simulink model "ABB_Samistar"  (R2020b)
settings: Solver=VariableStepAuto  StartTime=0.0  StopTime=50  RelTol=1e-3
model workspace (MAT data in the model file):
  KPS = Simulink.Parameter
  KPS.Value = 1
  KPS.DataType = 'auto'
  KPS.Dimensions = [1 1]
  KPU = Simulink.Parameter
  KPU.Value = 0.04
  KPU.DataType = 'auto'
  KPU.Dimensions = [1 1]
  P_dyn_ampl = Simulink.Parameter
  P_dyn_ampl.Value = 54
  P_dyn_ampl.DataType = 'auto'
  P_dyn_ampl.Dimensions = [1 1]
  P_dyn_slip = Simulink.Parameter
  P_dyn_slip.Value = 0.79333
  P_dyn_slip.DataType = 'auto'
  P_dyn_slip.Dimensions = [1 1]
  TIS = Simulink.Parameter
  TIS.Value = 1
  TIS.DataType = 'auto'
  TIS.Dimensions = [1 1]
  aantal_keer_freq_sinus = 30
  amplitude_sinus = 1
  freq_sinus = 50
  gewenste_ampitude_fasesp = 326
libraries: powerlib x12
settings Model: ParameterArgumentNames=KPU  OrderedModelArguments=off  Creator=Tijl J  LastModifiedBy=Tijl J
settings SolverCC: ZeroCrossAlgorithm=Adaptive  AlgebraicLoopSolver=LineSearch
settings DebuggingCC: IgnoredZcDiagnostic=none

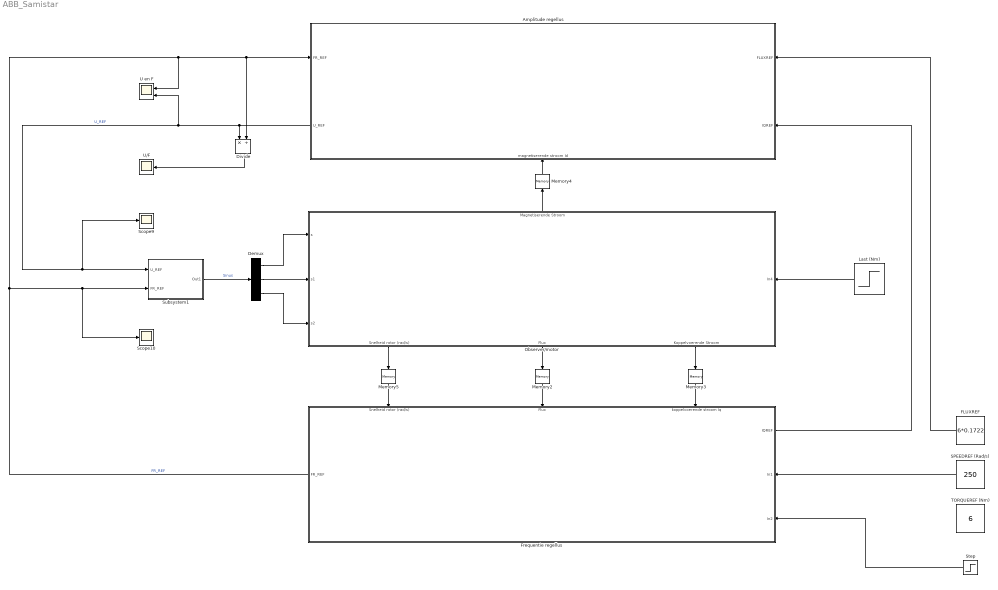
== system ABB_Samistar ==
  Amplitude regellus : Subsystem
      settings: PortSchema="{\"entries\":[{\"content\":{\"sides\":[{\"content\":{\"connectorIds\":[\"In1\",\"Out1\"]},\"type\":\"ConnectorPlacement.EquallySpacedRectSide\",\"uuid\":\"93bcf8db-9415-4baa-860c-11fdd531b56d\"},{\"content\":{\"connectorIds\":[\"In3\",\"In4\"],\"side\":\"RIGHT\"},\"type\":\"ConnectorPlacement.EquallySpacedRectSide\",\"uuid\":\"37029ce7-5e0f-4de3-a6e1-7a5c9d5a11f1\"},{\"content\":{\"connectorIds\":[],\"side\":\"TOP\"},\"type\":\"ConnectorPlacement.EquallySpacedRectSide\",\"uuid\":\"728afc0d-af0d-45f1-9722-28d57fd6c551\"},{\"content\":{\"connectorIds\":[\"In2\"],\"side\":\"BOTTOM\"},\"type\":\"ConnectorPlacement.EquallySpacedRectSide\",\"uuid\":\"07082ed3-f076-4bb5-ab11-0475c2dbd4ea\"}]},\"type\":\"ConnectorPlacement.EquallySpacedConnector\",\"uuid\":\"a9ce8458-6a15-4687-a7cd-fa30a873f563\"}],\"packageUris\":[\"http://schema.mathworks.com/mf0/Connector/19700101\"],\"version\":\"1.0\"}"
  Demux : Demux  Outputs=3
      settings: DisplayOption=none
  Divide : Product  Inputs=*/  RndMeth=Zero  SaturateOnIntegerOverflow=on
  FLUXREF : Constant  Value=6*0.1722
  Frequentie regellus : Subsystem
      settings: PortSchema="{\"entries\":[{\"content\":{\"sides\":[{\"content\":{\"connectorIds\":[\"Out2\"]},\"type\":\"ConnectorPlacement.EquallySpacedRectSide\",\"uuid\":\"9e8918ce-6ab1-4350-a27c-6c0740db8e36\"},{\"content\":{\"connectorIds\":[\"Out1\",\"In4\",\"In5\"],\"side\":\"RIGHT\"},\"type\":\"ConnectorPlacement.EquallySpacedRectSide\",\"uuid\":\"b7677f78-c4ce-4f8c-bcaa-757820ca5b4a\"},{\"content\":{\"connectorIds\":[\"In1\",\"In2\",\"In3\"],\"side\":\"TOP\"},\"type\":\"ConnectorPlacement.EquallySpacedRectSide\",\"uuid\":\"ce215d33-9ba4-4a26-b731-73f2d57ad5bf\"},{\"content\":{\"connectorIds\":[],\"side\":\"BOTTOM\"},\"type\":\"ConnectorPlacement.EquallySpacedRectSide\",\"uuid\":\"afaf8d9d-7f5b-47e6-9504-851e9c020fbe\"}]},\"type\":\"ConnectorPlacement.EquallySpacedConnector\",\"uuid\":\"a6238931-2ac8-4383-9bdd-f69522e27e3a\"}],\"packageUris\":[\"http://schema.mathworks.com/mf0/Connector/19700101\"],\"version\":\"1.0\"}"
  Last (Nm) : Step  Time=7  After=6  SampleTime=0
  Memory{2..5} (4 alike) : Memory
  Observer/motor : Subsystem
      settings: PortSchema="{\"entries\":[{\"content\":{\"sides\":[{\"content\":{\"connectorIds\":[\"In1\",\"In2\",\"In3\"]},\"type\":\"ConnectorPlacement.EquallySpacedRectSide\",\"uuid\":\"e974f17d-3e24-4aa3-9f71-ee26b6420732\"},{\"content\":{\"connectorIds\":[\"In4\"],\"side\":\"RIGHT\"},\"type\":\"ConnectorPlacement.EquallySpacedRectSide\",\"uuid\":\"7b407c95-e93c-432b-9353-b22fb20e7cb2\"},{\"content\":{\"connectorIds\":[\"Out4\"],\"side\":\"TOP\"},\"type\":\"ConnectorPlacement.EquallySpacedRectSide\",\"uuid\":\"82039074-d665-492a-9fb7-dc8321ceba23\"},{\"content\":{\"connectorIds\":[\"Out1\",\"Out2\",\"Out3\"],\"side\":\"BOTTOM\"},\"type\":\"ConnectorPlacement.EquallySpacedRectSide\",\"uuid\":\"28c56ceb-9a43-45d0-8e14-1b89590953e6\"}]},\"type\":\"ConnectorPlacement.EquallySpacedConnector\",\"uuid\":\"259d5e5a-eb05-4963-bbb5-562b18f45dd1\"}],\"packageUris\":[\"http://schema.mathworks.com/mf0/Connector/19700101\"],\"version\":\"1.0\"}"
  SPEEDREF (Rad/s) : Constant  Value=250
  Scope10 : Scope
  Scope9 : Scope
  Step : Step  Time=6  After=8  SampleTime=0
  Subsystem1 : Subsystem
  TORQUEREF (Nm) : Constant  Value=6
  U en F : Scope  NumInputPorts=2
  U/F : Scope
  wires:
  SPEEDREF (Rad/s)/1 -> Frequentie regellus/4(In1)
  FLUXREF/1 -> Amplitude regellus/3(FLUXREF)
  Frequentie regellus/1(IQREF) -> Amplitude regellus/4(IQREF)
  Amplitude regellus/1(U_REF) -> Scope9/1, Subsystem1/1(U_REF), U en F/2, Divide/1  "U_REF"
  Frequentie regellus/2(FR_REF) -> U en F/1, Amplitude regellus/1(FR_REF), Divide/2, Scope10/1, Subsystem1/2(FR_REF)  "FR_REF"
  Memory2/1 -> Frequentie regellus/2(Flux)
  Memory3/1 -> Frequentie regellus/3(koppelvoerende stroom Iq)
  Memory4/1 -> Amplitude regellus/2(magnetiserende stroom Id)
  Memory5/1 -> Frequentie regellus/1(Snelheid rotor (rad/s))
  Demux/1 -> Observer/motor/1(s)
  Demux/2 -> Observer/motor/2(s1)
  Demux/3 -> Observer/motor/3(s2)
  Observer/motor/4(Magnetiserende Stroom) -> Memory4/1
  Observer/motor/2(Flux) -> Memory2/1
  Observer/motor/1(Snelheid rotor (rad/s)) -> Memory5/1
  Observer/motor/3(Koppelvoerende Stroom) -> Memory3/1
  Subsystem1/1(Out1) -> Demux/1  "Sinus"
  Divide/1 -> U/F/1
  Last (Nm)/1 -> Observer/motor/4(In4)
  Step/1 -> Frequentie regellus/5(In2)

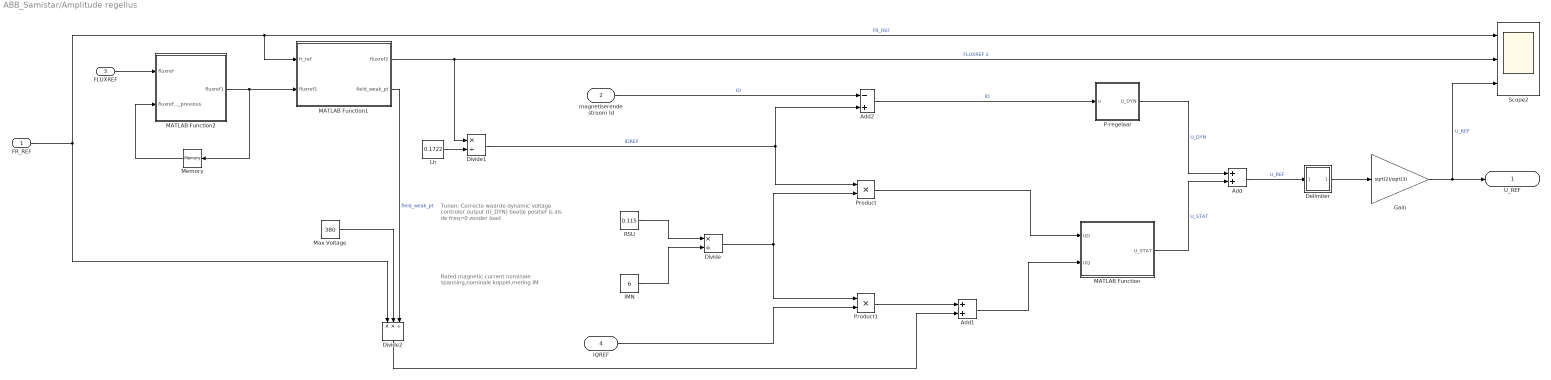
== system ABB_Samistar/Amplitude regellus ==
  note: Tunen:
      | Correcte waarde dynamic
      | voltage controler output (U_DYN)
      | beetje positief is als de freq=0 zonder load
  note: Rated magnetic current
      |
      | nominale spanning,nominale koppel,meting IM
  FR_REF : Inport
  magnetiserende stroom Id : Inport  Port=2
  FLUXREF : Inport  Port=3
  IQREF : Inport  Port=4
  Add : Sum
  Add1 : Sum
  Add2 : Sum  Inputs=-+
  Delimiter : MATLAB Function  TreatAsAtomicUnit=on
  Divide : Product  Inputs=*/
  Divide1 : Product  Inputs=*/
  Divide2 : Product  Inputs=**/
  Gain : Gain  Gain=sqrt(2)/sqrt(3)
  IMN : Constant  Value=6
  Lh : Constant  Value=0.1722
  MATLAB Function : MATLAB Function  TreatAsAtomicUnit=on
  MATLAB Function1 : MATLAB Function  TreatAsAtomicUnit=on  SystemSampleTime=0.001
  MATLAB Function2 : MATLAB Function  TreatAsAtomicUnit=on  SystemSampleTime=0.0001
  Max Voltage : Constant  Value=380
  Memory : Memory
  P-regelaar : Subsystem
  Product : Product
  Product1 : Product
  RSU : Constant  Value=0.115
  Scope2 : Scope  NumInputPorts=3
  U_REF : Outport
  wires:
  Add/1 -> Delimiter/1(U_REF_calculated)  "U_REF"
  MATLAB Function/1(U_STAT) -> Add/2  "U_STAT"
  Product/1 -> MATLAB Function/1(UD)
  Product1/1 -> Add1/1
  IQREF/1 -> Product1/2
  RSU/1 -> Divide/1
  IMN/1 -> Divide/2
  Divide/1 -> Product1/1, Product/2
  Add1/1 -> MATLAB Function/2(UQ)
  Divide2/1 -> Add1/2
  magnetiserende stroom Id/1 -> Add2/1  "ID"
  Divide1/1 -> Add2/2, Product/1  "IDREF"
  Add2/1 -> P-regelaar/1(u)  "ID"
  P-regelaar/1(U_DYN) -> Add/1  "U_DYN"
  MATLAB Function1/1(fluxref2) -> Divide1/1, Scope2/2  "FLUXREF 2"
  MATLAB Function2/1(fluxref1) -> Memory/1, MATLAB Function1/2(fluxref1)
  Memory/1 -> MATLAB Function2/2(fluxref1_previous)
  FR_REF/1 -> MATLAB Function1/1(fr_ref), Scope2/1, Divide2/1  "FR_REF"
  FLUXREF/1 -> MATLAB Function2/1(fluxref)
  MATLAB Function1/2(field_weak_pt) -> Divide2/3  "field_weak_pt"
  Max Voltage/1 -> Divide2/2
  Lh/1 -> Divide1/2
  Delimiter/1(U_REF) -> Gain/1
  Gain/1 -> U_REF/1, Scope2/3  "U_REF"

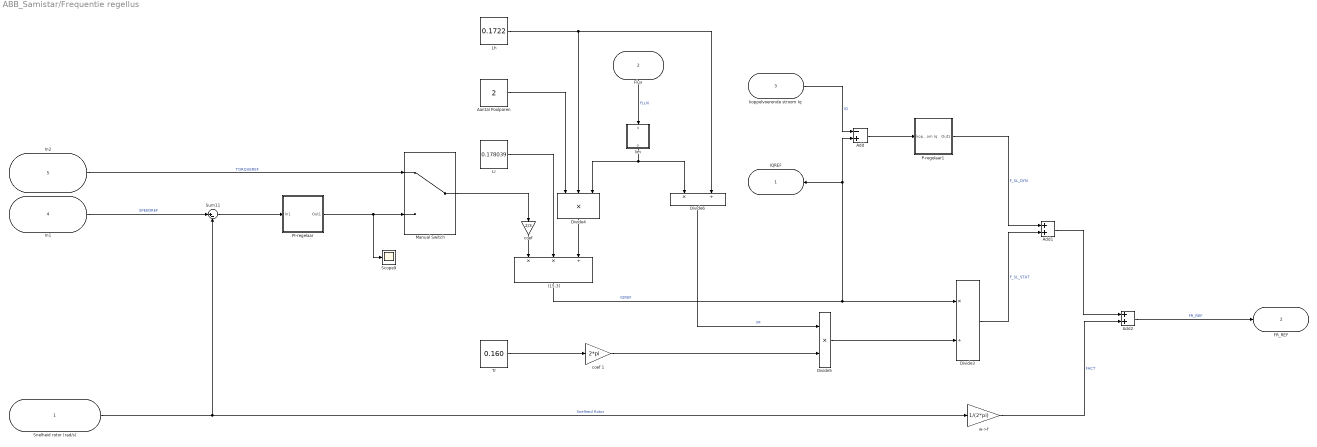
== system ABB_Samistar/Frequentie regellus ==
  Snelheid rotor (rad/s) : Inport
  Flux : Inport  Port=2
  koppelvoerende stroom Iq : Inport  Port=3
  In1 : Inport  Port=4
  In2 : Inport  Port=5
  (15.3) : Product  Inputs=**/
  Aantal Poolparen : Constant  Value=2
  Add : Sum  Inputs=-+
  Add1 : Sum
  Add2 : Sum
  Divide3 : Product  Inputs=*/
  Divide4 : Product  Inputs=***
  Divide5 : Product  Inputs=**
  Divide6 : Product  Inputs=*/
  Lh : Constant  Value=0.1722
  Lr : Constant  Value=0.178039
  Manual Switch : ManualSwitch
  P-regelaar1 : Subsystem
  PI-regelaar : Subsystem
  Scope9 : Scope
  Sum11 : Sum  Inputs=|+-
  Tr : Constant  Value=0.160
  "coef " : Gain  Gain=2/3
  coef 1 : Gain  Gain=2*pi
  lim : MATLAB Function  TreatAsAtomicUnit=on
  w->f : Gain  Gain=1/(2*pi)
  IQREF : Outport
  FR_REF : Outport  Port=2
  wires:
  Lh/1 -> Divide4/2, Divide6/2
  Divide4/1 -> (15.3)/3
  Aantal Poolparen/1 -> Divide4/1
  In2/1 -> Manual Switch/1  "TORQUEREF"
  Snelheid rotor (rad/s)/1 -> Sum11/2, w->f/1  "Snelheid Rotor"
  coef 1/1 -> Divide5/2
  Divide3/1 -> Add1/2  "F_SL_STAT"
  Sum11/1 -> PI-regelaar/1(In1)
  (15.3)/1 -> Add/2, IQREF/1, Divide3/1  "IQREF"
  PI-regelaar/1(Out1) -> Scope9/1, Manual Switch/2
  Flux/1 -> lim/1(u)  "FLUX"
  "coef "/1 -> (15.3)/1
  Add2/1 -> FR_REF/1  "FR_REF"
  Divide6/1 -> Divide5/1  "IM"
  Manual Switch/1 -> "coef "/1
  Tr/1 -> coef 1/1
  w->f/1 -> Add2/2  "FACT"
  P-regelaar1/1(Out1) -> Add1/1  "F_SL_DYN"
  Divide5/1 -> Divide3/2
  koppelvoerende stroom Iq/1 -> Add/1  "IQ"
  In1/1 -> Sum11/1  "SPEEDREF"
  Add/1 -> P-regelaar1/1(koppelvoerende stroom Iq)
  Lr/1 -> (15.3)/2
  lim/1(y) -> Divide6/1, Divide4/3
  Add1/1 -> Add2/1

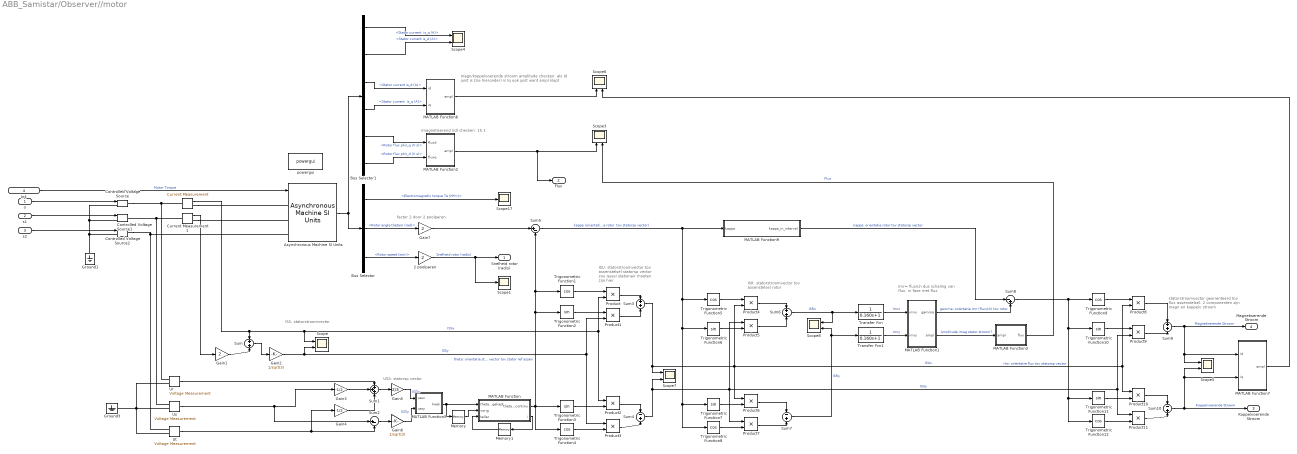
== system ABB_Samistar/Observer//motor ==
  note: Imagnetiserend (id) checken: 15.1
  note: magn/koppelvoerende stroom amplitude checken:
      | als Id juist is (zie hieronder) is Iq ook juist want ampl
      | klopt
  note: ISS: statorstroomvector
  note: USS: statorsp vector
  note: statorstroomvector georienteerd
      | tov flux assenstelsel: 2 componenten
      | zijn magn en koppelv stroom
  note: Imr= flux/Lh dus schaling
      | van flux, in fase met flux
  note: ISU: statorstroomvector tov
      | assenstelsel statorsp vector
      | zou quasi stationair moeten
      | zijn hier
  note: ISR: statorstroomvector tov
      | assenstelsel rotor
  note: factor 2 door 2 poolparen
  s : Inport
  s1 : Inport  Port=2
  s2 : Inport  Port=3
  In4 : Inport  Port=4
  " " : powerlib/Measurements/Current Measurement  PhasorSimulation=off  OutputType=Complex  PSBequivalent=0
  2 poolparen : Gain  Gain=2
  Asynchronous Machine SI Units : powerlib/Machines/Asynchronous Machine SI Units  RotorType=Squirrel-cage  PresetModel="15:  5.4 HP (4KW)   400 V  50Hz 1430 RPM"  MechanicalLoad=Torque Tm  ShowDetailedParameters=on  ReferenceFrame=Synchronous  Units=SI  MeasurementBus=off  NominalParameters=[4000 400 50]  Stator=[1.405 0.005839]  Rotor=[1.395 0.005839]  Cage1=[0.4155 0.002066]  Cage2=[0.4168 0.0003495]  Lm=0.1722  Mechanical=[0.0131 0.002985 2]  PolePairs=2  InitialConditions=[0 0 0 0 0 0 0 0]  SimulateSaturation=off  Saturation=[14.03593122, 27.81365428, 53.79336849, 68, 82, 96, 110,124, 130 ; 230, 322, 414, 460, 506, 552, 598, 644, 690]  LoadFlowParameters=1492000  TsPowergui=0  TsBlock=-1  IterativeModel=Trapezoidal non iterative  IterativeDiscreteModel=Trapezoidal non iterative  Pmec=1.492e+006
  Bus Selector : BusSelector  OutputSignals=Mechanical.Electromagnetic torque Te (N*m),Mechanical.Rotor angle thetam (rad),Mechanical.Rotor speed (wm)
  Bus Selector1 : BusSelector  OutputSignals="Stator measurements.Stator current  is_q (A),Stator measurements.Stator current is_d (A),Stator measurements.Stator current is_d (A),Stator measurements.Stator current  is_q (A),Rotor measurements.Rotor flux phir_q (V s),Rotor measurements.Rotor flux phir_d (V s)"
  Controlled Voltage Source : powerlib/Electrical Sources/Controlled Voltage Source  Initialize=on  Source_Type=AC  Amplitude=0  Phase=0  Frequency=0  Measurements=None
  Controlled Voltage Source1 : powerlib/Electrical Sources/Controlled Voltage Source  Initialize=on  Source_Type=AC  Amplitude=0  Phase=0  Frequency=0  Measurements=None
  Controlled Voltage Source2 : powerlib/Electrical Sources/Controlled Voltage Source  Initialize=on  Source_Type=AC  Amplitude=0  Phase=0  Frequency=0  Measurements=None
  Current Measurement1 : powerlib/Measurements/Current Measurement  PhasorSimulation=off  OutputType=Complex  PSBequivalent=0
  Gain1 : Gain  Gain=2
  Gain2 : Gain  Gain=1/sqrt(3)
  Gain3 : Gain  Gain=-1/2
  Gain4 : Gain  Gain=-1/2
  Gain5 : Gain  Gain=2/3
  Gain6 : Gain  Gain=1/sqrt(3)
  Gain7 : Gain  Gain=2
  Ground1 : powerlib/Elements/Ground  LConnTagsString=a
  Ground3 : powerlib/Elements/Ground  LConnTagsString=a
  MATLAB Function : MATLAB Function  TreatAsAtomicUnit=on
  MATLAB Function1 : MATLAB Function  TreatAsAtomicUnit=on
  MATLAB Function2 : MATLAB Function  TreatAsAtomicUnit=on
  MATLAB Function3 : MATLAB Function  TreatAsAtomicUnit=on
  MATLAB Function5 : MATLAB Function  TreatAsAtomicUnit=on
  MATLAB Function6 : MATLAB Function  TreatAsAtomicUnit=on
  MATLAB Function7 : MATLAB Function  TreatAsAtomicUnit=on
  MATLAB Function9 : MATLAB Function  TreatAsAtomicUnit=on
  Memory : Memory
  Memory1 : Memory
  Product{,1..11} (12 alike) : Product
  Scope{,3..8} (7 alike) : Scope  NumInputPorts=2
  Scope1 : Scope
  Scope17 : Scope
  Sum : Sum
  Sum1 : Sum  Inputs=3
  Sum10 : Sum  Inputs=-+
  Sum2 : Sum  Inputs=|+-
  Sum3 : Sum  Inputs=2
  Sum4 : Sum  Inputs=-+
  Sum5 : Sum  Inputs=|+-
  Sum6 : Sum
  Sum7 : Sum  Inputs=-+
  Sum8 : Sum  Inputs=|-+
  Sum9 : Sum
  Transfer Fcn : TransferFcn  Denominator=[0.160 1]
  Transfer Fcn1 : TransferFcn  Denominator=[0.160 1]
  Trigonometric Function{1,4..5,8..9,12} (6 alike) : Trigonometry  Operator=cos
  Trigonometric Function{2..3,6..7,10..11} (6 alike) : Trigonometry
  Ur : powerlib/Measurements/Voltage Measurement  PhasorSimulation=off  OutputType=Complex  PSBequivalent=0
  Us : powerlib/Measurements/Voltage Measurement  PhasorSimulation=off  OutputType=Complex  PSBequivalent=0
  Ut : powerlib/Measurements/Voltage Measurement  PhasorSimulation=off  OutputType=Complex  PSBequivalent=0
  powergui : powerlib/powergui  Priority=1  SimulationMode=Continuous  SampleTime=50e-6  frequency=60  Iterations=50  frequencyindice=50  Pbase=100e6  ErrMax=1e-4  UnitsV=kV  UnitsW=MW  buscounter=0  FunctionMessages=off  echomessages=off  EnableUseOfTLC=off  CurrentSourceSwitches=off  DisableSnubberDevices=off  DisableRonSwitches=off  DisableVfSwitches=off  DisplayEquations=off  AutomaticDiscreteSolvers=off  SolverType=Tustin/Backward Euler (TBE)  Interpol=off  ExternalGateDelay=off  methode=off  Ts=100  x0status=blocks  SPID=on  SwTol=0  HookPort=off  NonlinearTolerance=1e-4  nMaxIteration=100  ContinueOnMaxIteration=off  RestoreLinks=warning  ResistiveCurrentMeasurement=off  Frange=[0:2:500]  Ylog=off  Xlog=on  ShowGrid=off  save=off  variable=ZData  structure=0  ZoomFFT=off  StartTime=0.0  cycles=1  DisplayStyle=1  fundamental=60  FreqAxis=off  MaxFrequency=1000  frequencyindicesteady=1  RmsSteady=1  display=off
  Snelheid rotor (rad/s) : Outport
  Flux : Outport  Port=2
  Koppelvoerende Stroom : Outport  Port=3
  Magnetiserende Stroom : Outport  Port=4
  wires:
  Gain1/1 -> Sum/2
  Trigonometric Function8/1 -> Product7/2
  Ur/1 -> Sum1/1
  Product3/1 -> Sum4/2
  Bus Selector1/2 -> Scope4/2  "<Stator current is_d (A)>"
  Bus Selector/2 -> Gain7/1  "<Rotor angle thetam (rad)>"
  Asynchronous Machine SI Units/1 -> Bus Selector1/1, Bus Selector/1
  Bus Selector1/1 -> Scope4/1  "<Stator current  is_q (A)>"
  Us/1 -> Gain3/1, Sum2/1
  Sum8/1 -> Trigonometric Function12/1, Trigonometric Function11/1, Trigonometric Function10/1, Trigonometric Function9/1  "rho: oriëntatie flux tov statorsp vector"
  MATLAB Function/1(theta_continu) -> Trigonometric Function4/1, Trigonometric Function1/1, Sum5/2, Trigonometric Function2/1, Trigonometric Function3/1  "theta: orientatie stator sp vector tov stator ref assen"
  Product5/1 -> Sum6/2
  Trigonometric Function7/1 -> Product6/2
  s/1 -> Controlled Voltage Source/1
  Sum10/1 -> Scope5/2, MATLAB Function7/2(iq), Koppelvoerende Stroom/1  "Koppelvoerende Stroom"
  Sum4/1 -> Product11/1, Product9/2, Product5/1, Product7/1, Scope7/2  "ISUy"
  Trigonometric Function4/1 -> Product3/2
  Ut/1 -> Gain4/1, Sum2/2
  MATLAB Function2/1(ampl) -> Flux/1, Scope3/1
  Sum3/1 -> Product8/2, Product10/1, Product4/2, Product6/1, Scope7/1  "ISUx"
  Sum/1 -> Gain2/1
  Current Measurement1/1 -> Gain1/1
  Sum5/1 -> MATLAB Function9/1(kappa), Trigonometric Function8/1, Trigonometric Function7/1, Trigonometric Function6/1, Trigonometric Function5/1  "kappa (orientatie rotor  tov statorsp vector)"
  Trigonometric Function9/1 -> Product8/1
  MATLAB Function5/1(hoek) -> Memory/1, MATLAB Function/1(theta_gekapt)
  Sum1/1 -> Gain5/1
  Gain4/1 -> Sum1/3
  Gain7/1 -> Sum5/1
  Trigonometric Function2/1 -> Product1/1
  Product4/1 -> Sum6/1
  Gain5/1 -> MATLAB Function5/1(ussx)  "USSx"
  Product7/1 -> Sum7/2
  s2/1 -> Controlled Voltage Source2/1
  Sum2/1 -> Gain6/1
  Sum9/1 -> Scope5/1, MATLAB Function7/1(id), Magnetiserende Stroom/1  "Magnetiserende Stroom"
  MATLAB Function7/1(ampl) -> Scope6/2
  Sum6/1 -> Scope8/1, Transfer Fcn/1  "ISRx"
  MATLAB Function9/1(kappa_in_interval) -> Sum8/1  "kappa: orientatie rotor tov statorsp vector"
  Product/1 -> Sum3/1
  s1/1 -> Controlled Voltage Source1/1
  Trigonometric Function3/1 -> Product2/2
  Product1/1 -> Sum3/2
  2 poolparen/1 -> Scope1/1, Snelheid rotor (rad/s)/1  "Snelheid rotor (rad/s)"
  " "/1 -> Sum/1, Scope/1, Product/2, Product2/1  "ISSx"
  Gain2/1 -> Scope/2, Product1/2, Product3/1  "ISSy"
  MATLAB Function1/2(ampl) -> MATLAB Function3/1(ampl)  "Amplitude imag stator stroom?"
  Trigonometric Function6/1 -> Product5/2
  Product6/1 -> Sum7/1
  Gain6/1 -> MATLAB Function5/2(ussy)  "USSy"
  Trigonometric Function5/1 -> Product4/1
  Bus Selector/1 -> Scope17/1  "<Electromagnetic torque Te (N*m)>"
  Product2/1 -> Sum4/1
  Memory/1 -> MATLAB Function/2(vorig)
  Memory1/1 -> MATLAB Function/3(teller)
  MATLAB Function/2(i) -> Memory1/1
  Trigonometric Function10/1 -> Product9/1
  Sum7/1 -> Scope8/2, Transfer Fcn1/1  "ISRy"
  Product10/1 -> Sum10/1
  Product9/1 -> Sum9/2
  Trigonometric Function12/1 -> Product11/2
  Gain3/1 -> Sum1/2
  Trigonometric Function11/1 -> Product10/2
  Transfer Fcn/1 -> MATLAB Function1/1(imrx)  "Imrx"
  MATLAB Function1/1(gamma) -> Sum8/2  "gamma: oriëntatie Imr (flux/Lh) tov rotor"
  Bus Selector1/5 -> MATLAB Function2/1(fluxd)  "<Rotor flux phir_q (V s)>"
  Bus Selector1/3 -> MATLAB Function6/1(id)  "<Stator current is_d (A)>"
  Product8/1 -> Sum9/1
  MATLAB Function6/1(ampl) -> Scope6/1
  MATLAB Function3/1(flux) -> Scope3/2  "Flux"
  Trigonometric Function1/1 -> Product/1
  Bus Selector/3 -> 2 poolparen/1  "<Rotor speed (wm)>"
  Bus Selector1/4 -> MATLAB Function6/2(iq)  "<Stator current  is_q (A)>"
  Transfer Fcn1/1 -> MATLAB Function1/2(imry)  "Imry"
  Product11/1 -> Sum10/2
  Bus Selector1/6 -> MATLAB Function2/2(fluxq)  "<Rotor flux phir_d (V s)>"
  In4/1 -> Asynchronous Machine SI Units/1  "Motor Torque"
  connections:
  Ut/LConn2 -- Ur/LConn2 -- Us/LConn2 -- Ground3/LConn1
  Controlled Voltage Source/RConn1 -- Ur/LConn1 -- " "/LConn1
  " "/RConn1 -- Asynchronous Machine SI Units/LConn1
  Current Measurement1/RConn1 -- Asynchronous Machine SI Units/LConn2
  Current Measurement1/LConn1 -- Us/LConn1 -- Controlled Voltage Source1/RConn1
  Controlled Voltage Source1/LConn1 -- Controlled Voltage Source2/LConn1 -- Ground1/LConn1 -- Controlled Voltage Source/LConn1
  Ut/LConn1 -- Controlled Voltage Source2/RConn1 -- Asynchronous Machine SI Units/LConn3

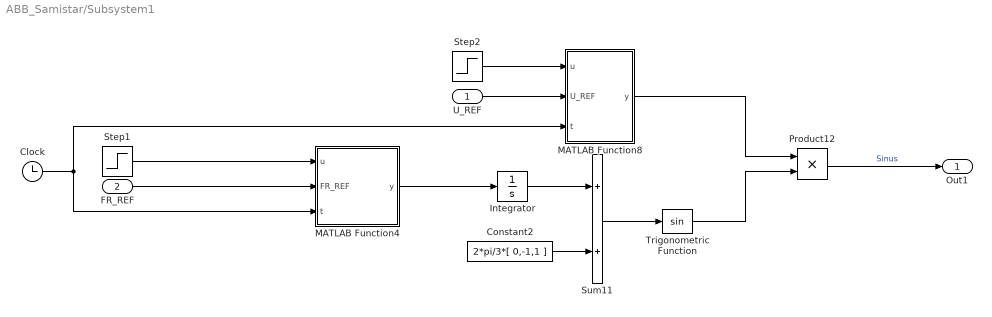
== system ABB_Samistar/Subsystem1 ==
  U_REF : Inport
  FR_REF : Inport  Port=2
  Clock : Clock
  Constant2 : Constant  Value=2*pi/3*[ 0,-1,1 ]
  Integrator : Integrator
  MATLAB Function4 : MATLAB Function  TreatAsAtomicUnit=on
  MATLAB Function8 : MATLAB Function  TreatAsAtomicUnit=on
  Product12 : Product
  Step1 : Step  Time=0  After=50  SampleTime=0
  Step2 : Step  Time=0  After=326  SampleTime=0
  Sum11 : Sum  InputSameDT=on  SaturateOnIntegerOverflow=on  OutDataTypeStr=Inherit: Same as first input
  Trigonometric Function : Trigonometry
  Out1 : Outport
  wires:
  Clock/1 -> MATLAB Function8/3(t), MATLAB Function4/3(t)
  U_REF/1 -> MATLAB Function8/2(U_REF)
  Trigonometric Function/1 -> Product12/2
  Step1/1 -> MATLAB Function4/1(u)
  Constant2/1 -> Sum11/2
  MATLAB Function4/1(y) -> Integrator/1
  MATLAB Function8/1(y) -> Product12/1
  Step2/1 -> MATLAB Function8/1(u)
  Sum11/1 -> Trigonometric Function/1
  Integrator/1 -> Sum11/1
  Product12/1 -> Out1/1  "Sinus"
  FR_REF/1 -> MATLAB Function4/2(FR_REF)

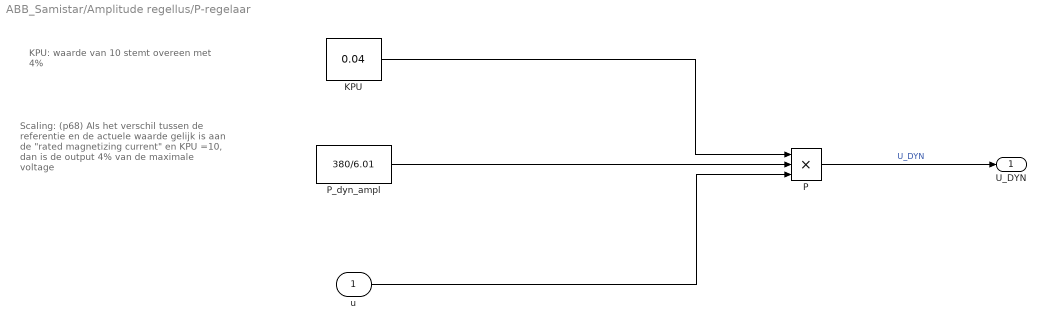
== system ABB_Samistar/Amplitude regellus/P-regelaar ==
  note: KPU:
      | waarde van 10 stemt overeen met 4%
  note: Scaling: (p68)
      |
      | Als het verschil tussen de referentie en de actuele waarde gelijk is aan de "rated magnetizing current" en KPU =10, dan is de output 4% van de maximale voltage
  u : Inport
  KPU : Constant  Value=0.04
  "P " : Product  Inputs=3
  P_dyn_ampl : Constant  Value=380/6.01
  U_DYN : Outport
  wires:
  "P "/1 -> U_DYN/1  "U_DYN"
  u/1 -> "P "/3
  KPU/1 -> "P "/1
  P_dyn_ampl/1 -> "P "/2

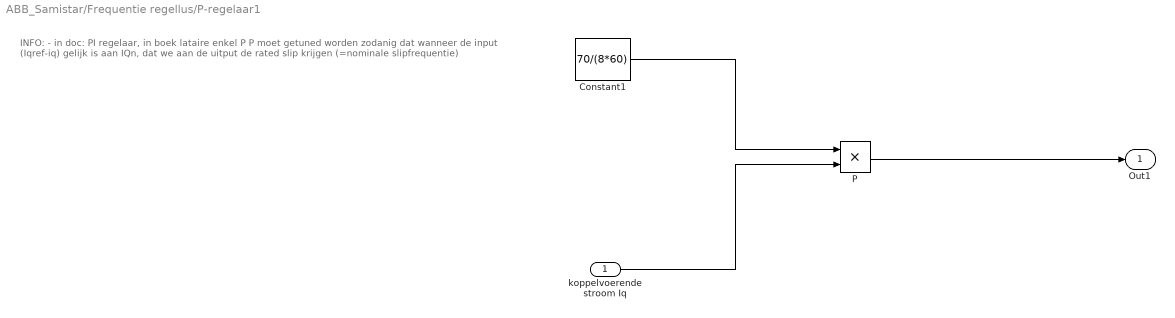
== system ABB_Samistar/Frequentie regellus/P-regelaar1 ==
  note: INFO:
      |
      | - in doc: PI regelaar, in boek lataire enkel P
      |
      | P moet getuned worden zodanig dat
      | wanneer de input (Iqref-iq) gelijk is aan IQn,
      | dat we aan de uitput de rated slip krijgen
      | (=nominale slipfrequentie)
  koppelvoerende stroom Iq : Inport
  Constant1 : Constant  Value=70/(8*60)
  "P " : Product
  Out1 : Outport
  wires:
  koppelvoerende stroom Iq/1 -> "P "/2
  "P "/1 -> Out1/1
  Constant1/1 -> "P "/1

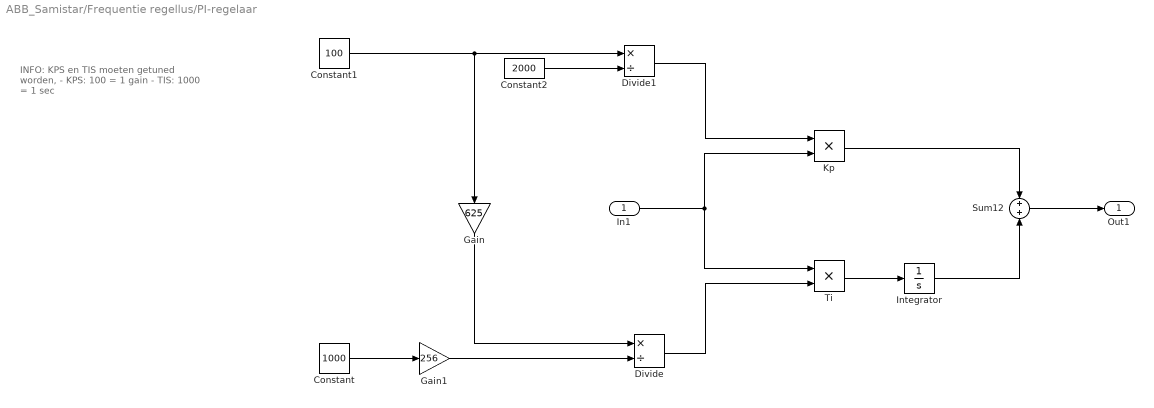
== system ABB_Samistar/Frequentie regellus/PI-regelaar ==
  note: INFO:
      |
      | KPS en TIS moeten getuned worden,
      |
      | - KPS: 100 = 1 gain
      | - TIS: 1000 = 1 sec
  In1 : Inport
  Constant : Constant  Value=1000
  Constant1 : Constant  Value=100
  Constant2 : Constant  Value=2000
  Divide : Product  Inputs=*/
  Divide1 : Product  Inputs=*/
  Gain : Gain  Gain=625
  Gain1 : Gain  Gain=256
  Integrator : Integrator
  Kp : Product
  Sum12 : Sum
  Ti : Product
  Out1 : Outport
  wires:
  Ti/1 -> Integrator/1
  Kp/1 -> Sum12/1
  In1/1 -> Ti/1, Kp/2
  Integrator/1 -> Sum12/2
  Sum12/1 -> Out1/1
  Divide/1 -> Ti/2
  Divide1/1 -> Kp/1
  Constant1/1 -> Gain/1, Divide1/1
  Constant2/1 -> Divide1/2
  Gain/1 -> Divide/1
  Constant/1 -> Gain1/1
  Gain1/1 -> Divide/2

== matlab function ABB_Samistar/Observer//motor/MATLAB Function1 ==
  data: gamma output; imrx input; ampl output; imry input
function [gamma,ampl] = fcn(imrx,imry)
ampl = sqrt(imrx^2+imry^2);
gamma = atan2(imry,imrx); %% geeft radialen weer
end

== matlab function ABB_Samistar/Amplitude regellus/MATLAB Function2 ==
  data: fluxref input; fluxref1 output; fluxref1_previous input
function fluxref1 = hellingsbegrenzer(fluxref,fluxref1_previous)
%dit blokje staat op een vaste sample time van 0.001, zal dus 1000 keer per
%seconde dit uitvoeren, aan te passen door rechtermuisklik op blokje -> 
%block parameters (subsystem) -> sample time op 0.001 gezet, default op -1

dt=0.001; %zodat er geen timer moet gebruikt worden
max_slope=0.1; %helling van 1000 per seconde, wlh jsp
fluxref1_init=0;
if isempty(fluxref1_previous)
    fluxref1_previous=fluxref1_init; %je moet een beginwaarde hebben anders da gaat ni
end
    
fluxref1=fluxref1_previous;

if fluxref>fluxref1_previous
    fluxref1=fluxref1+max_slope*dt;
elseif fluxref<fluxref1_previous
    fluxref1=fluxref1-max_slope*dt;
end
end

== matlab function ABB_Samistar/Frequentie regellus/lim ==
  data: u input; y output
function y = delimiter(u)
if u<0.05
    y=0.05;
else
    y=u;
end
end

== matlab function ABB_Samistar/Subsystem1/MATLAB Function8 ==
  data: u input; y output; U_REF input; t input
function y = fcn(u, U_REF, t)
if t<0.1
   y=u;
else
    y=U_REF;
end

== matlab function ABB_Samistar/Amplitude regellus/Delimiter ==
  data: U_REF_calculated input; U_REF output
function U_REF= fcn(U_REF_calculated)
if U_REF_calculated>380
    U_REF=380;
else
    U_REF=U_REF_calculated;
end

== matlab function ABB_Samistar/Observer//motor/MATLAB Function ==
  data: theta_gekapt input; theta_continu output; vorig input; teller input; i output
function [theta_continu,i] = fcn(theta_gekapt,vorig,teller)
i=teller;
if isempty(vorig)
   theta_continu=theta_gekapt ;
else
    if theta_gekapt<0 && vorig>0
        i=teller+1;
    end
    theta_continu=theta_gekapt+i*2*pi;    
end
end

== matlab function ABB_Samistar/Observer//motor/MATLAB Function2 ==
  data: fluxd input; ampl output; fluxq input
function ampl  = fcn(fluxd,fluxq)
ampl = sqrt(fluxd^2+fluxq^2);
end

== matlab function ABB_Samistar/Observer//motor/MATLAB Function3 ==
  data: ampl input; flux output
function flux = fcn(ampl)

flux = 0.1722 * ampl; % met verzadiging wordt deze formule ingewikkelder

== matlab function ABB_Samistar/Subsystem1/MATLAB Function4 ==
  data: u input; y output; FR_REF input; t input
function y = fcn(u, FR_REF, t)
if t<0.1
   y=u*2*pi;
else
    y=FR_REF*2*pi;
end

== matlab function ABB_Samistar/Observer//motor/MATLAB Function5 ==
  data: ussx input; hoek output; ussy input
function hoek = fcn(ussx,ussy)

hoek = atan2(ussy,ussx);
end

== matlab function ABB_Samistar/Observer//motor/MATLAB Function6 ==
  data: id input; ampl output; iq input
function ampl  = fcn(id,iq)
ampl = sqrt(id^2+iq^2);
end

== matlab function ABB_Samistar/Observer//motor/MATLAB Function7 ==
  data: id input; ampl output; iq input
function ampl  = fcn(id,iq)
ampl = sqrt(id^2+iq^2);
end

== matlab function ABB_Samistar/Amplitude regellus/MATLAB Function ==
  data: UD input; UQ input; U_STAT output
function U_STAT  = fcn(UD,UQ)

U_STAT = sqrt(UD^2+UQ^2);

== matlab function ABB_Samistar/Observer//motor/MATLAB Function9 ==
  data: kappa input; kappa_in_interval output
function kappa_in_interval = fcn(kappa)
if kappa> -pi &&kappa<pi
    kappa_in_interval=-kappa;
    
else

    kappa_in_interval=-(mod(kappa-pi,2*pi)-pi);

end
end

== matlab function ABB_Samistar/Amplitude regellus/MATLAB Function1 ==
  data: fr_ref input; fluxref1 input; fluxref2 output; field_weak_pt output
function [fluxref2,field_weak_pt] = blokje20(fr_ref,fluxref1)    
%dit blokje wordt ook fixed 1000 keer per seconde uitgevoerd, aan te passen
%door rechtermuisklik op blokje -> block parameters (subsystem) -> sample
%time op 0.001 gezet, default op -1

%karakteristieken motor
nom_freq=50; 
nom_voltage=400;
%aangelegde sinussen, normaal cst voltage
aangelegd_voltage=380;

field_weak_pt=nom_freq/nom_voltage*aangelegd_voltage; %mocht initieel constant verondersteld worden



if fr_ref<=field_weak_pt
    fluxref2 = fluxref1;
else
    cst=fluxref1*field_weak_pt;
    fluxref2=cst/fr_ref;
end
end
